simulink model "Sim_q3"  (Simulink 9.1)
settings: Solver=ode45  StartTime=0.0  StopTime=Tend  MaxStep=dt  RelTol=1e-3  EnableMultiTasking=on
InitFcn:
  | dt=1/100;
StopFcn:
  | close all;
  | t=Dados.time;
  | ref=Dados.signals.values(:,1);
  | es=Dados.signals.values(:,2);
  | y=Dados.signals.values(:,3);
  | ys=Dados.signals.values(:,4);
  | plot(t,ref,'k-',t,y,'r-'); hold on;
  | stairs(t,ys,'b-');
  | xlabel('t (s)');
  | legend('Ref(t)','Y(t)','Ys(t)');
  | title(['T = ', num2str(T), ' s']);
  | grid;
values from neighbouring files (symbols this model uses):
  T = 0.02589    [q6.m]
undefined symbols (not defined in the file or in its folder): Fref, w
settings Model: Creator=cairo  LastModifiedBy=Avell
settings DataIOCC: LimitDataPoints=on  SignalLoggingSaveFormat=ModelDataLogs
settings OptimizationCC: ExpressionDepthLimit=2147483647
settings DebuggingCC: SolverPrmCheckMsg=warning  FcnCallInpInsideContextMsg=warning  StateNameClashWarn=warning
settings GRTTargetCC: GeneratePreprocessorConditionals=Disable all

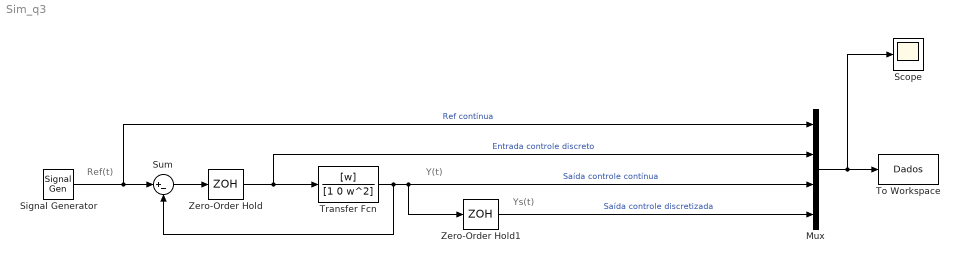
== system Sim_q3 ==
  note: Ref(t)
  note: Y(t)
  note: Ys(t)
  Mux : Mux
  Scope : Scope
  Signal Generator : SignalGenerator  WaveForm=square  Frequency=Fref
  Sum : Sum  Inputs=|+-
  To Workspace : ToWorkspace  VariableName=Dados  SaveFormat=Structure With Time  SampleTime=-1
  Transfer Fcn : TransferFcn  Numerator=[w]  Denominator=[1 0 w^2]
  Zero-Order Hold : ZeroOrderHold  SampleTime=T
  Zero-Order Hold1 : ZeroOrderHold  SampleTime=T
  wires:
  Signal Generator/1 -> Sum/1, Mux/1  "Ref contínua"
  Sum/1 -> Zero-Order Hold/1
  Zero-Order Hold/1 -> Transfer Fcn/1, Mux/2  "Entrada controle discreto"
  Transfer Fcn/1 -> Sum/2, Mux/3, Zero-Order Hold1/1  "Saída controle contínua"
  Mux/1 -> Scope/1, To Workspace/1
  Zero-Order Hold1/1 -> Mux/4  "Saída controle discretizada"
